simulink library "HEMERO"  (Simulink 3.00)
values from neighbouring files (symbols this model uses):
  K1 = 0.5    [ejh64.m]    (also in ejh65.m)
  K2 = 0.8    [ejh64.m]    (also in ejh65.m)
  x_camino = 0:0.01:10    [ejh64.m]    (also in ejh65.m)
  y_camino = x_camino.^2    [ejh64.m]    (also in ejh65.m)
undefined symbols (not defined in the file or in its folder): magnitude, nonlinear
libraries: simulink_extras x12, HEMERO x9, simulink3 x6, dspstat x4
(part 9 of 9)

== system HEMERO/Robots móviles/Control de robots móviles/Métodos basados en Teoría de Control/Seguimiento de caminos/Ejemplos/Ejemplo H.6.4/Seguimiento de caminos (control lineal)/Cálculo de parámetros/Subsystem/Parametros de Curvatura/coordenada x c. curvatura ==
  x_1 : Inport  Port=1  PortWidth=-1  SampleTime=-1  DataType=auto
      settings: SignalType=auto
  x_2 : Inport  Port=2  PortWidth=-1  SampleTime=-1  DataType=auto
      settings: SignalType=auto
  x_3 : Inport  Port=3  PortWidth=-1  SampleTime=-1  DataType=auto
      settings: SignalType=auto
  y_1 : Inport  Port=4  PortWidth=-1  SampleTime=-1  DataType=auto
      settings: SignalType=auto
  y_2 : Inport  Port=5  PortWidth=-1  SampleTime=-1  DataType=auto
      settings: SignalType=auto
  y_3 : Inport  Port=6  PortWidth=-1  SampleTime=-1  DataType=auto
      settings: SignalType=auto
  Constant : Constant  Value=0.00000001
  Math Function : Math  Operator=reciprocal  OutputSignalType=auto
  Product{,1..4} (5 alike) : Product  Inputs=2  SaturateOnIntegerOverflow=on
  Sum : Sum  Inputs=+-  SaturateOnIntegerOverflow=on
  Sum1 : Sum  Inputs=+-  SaturateOnIntegerOverflow=on
  Switch : Switch  Threshold=0.00000001
  bloque_1 : Subsystem
  bloque_2 : Subsystem
  x_g : Outport  Port=1  InitialOutput=0
  wires:
  Switch/1 -> Math Function/1
  Constant/1 -> Switch/3
  Sum1/1 -> Switch/1, Switch/2
  Product4/1 -> x_g/1
  Product/1 -> Sum/1
  Product1/1 -> Sum/2
  Product2/1 -> Sum1/1
  Product3/1 -> Sum1/2
  Math Function/1 -> Product4/2
  bloque_1/3(c_1) -> Product/2
  bloque_2/3(c_2) -> Product1/2
  bloque_2/2(beta_2) -> Product/1, Product2/2
  bloque_1/1(alfa_1) -> Product2/1
  bloque_1/2(beta_1) -> Product1/1, Product3/1
  bloque_2/1(alfa_2) -> Product3/2
  x_1/1 -> bloque_1/1(x1)
  x_2/1 -> bloque_1/2(x2), bloque_2/1(x2)
  y_1/1 -> bloque_1/3(y1)
  x_3/1 -> bloque_2/2(x3)
  y_2/1 -> bloque_2/3(y2), bloque_1/4(y2)
  y_3/1 -> bloque_2/4(y3)
  Sum/1 -> Product4/1

== system HEMERO/Robots móviles/Control de robots móviles/Métodos basados en Teoría de Control/Seguimiento de caminos/Ejemplos/Ejemplo H.6.4/Seguimiento de caminos (control lineal)/Cálculo de parámetros/Subsystem/Parametros de Curvatura/coordenada y c. curvatura ==
  x_1 : Inport  Port=1  PortWidth=-1  SampleTime=-1  DataType=auto
      settings: SignalType=auto
  x_2 : Inport  Port=2  PortWidth=-1  SampleTime=-1  DataType=auto
      settings: SignalType=auto
  x_3 : Inport  Port=3  PortWidth=-1  SampleTime=-1  DataType=auto
      settings: SignalType=auto
  y_1 : Inport  Port=4  PortWidth=-1  SampleTime=-1  DataType=auto
      settings: SignalType=auto
  y_2 : Inport  Port=5  PortWidth=-1  SampleTime=-1  DataType=auto
      settings: SignalType=auto
  y_3 : Inport  Port=6  PortWidth=-1  SampleTime=-1  DataType=auto
      settings: SignalType=auto
  Constant : Constant  Value=0.00000001
  Math Function : Math  Operator=reciprocal  OutputSignalType=auto
  Product{,1..4} (5 alike) : Product  Inputs=2  SaturateOnIntegerOverflow=on
  Sum : Sum  Inputs=+-  SaturateOnIntegerOverflow=on
  Sum1 : Sum  Inputs=+-  SaturateOnIntegerOverflow=on
  Switch : Switch  Threshold=0.00000001
  bloque_1 : Subsystem
  bloque_2 : Subsystem
  y_g : Outport  Port=1  InitialOutput=0
  wires:
  Constant/1 -> Switch/3
  Sum1/1 -> Switch/1, Switch/2
  Switch/1 -> Math Function/1
  Math Function/1 -> Product4/2
  Product4/1 -> y_g/1
  bloque_2/3(c_2) -> Product/2
  bloque_1/3(c_1) -> Product1/1
  bloque_1/1(alfa_1) -> Product/1, Product2/1
  bloque_2/2(beta_2) -> Product2/2
  bloque_1/2(beta_1) -> Product3/2
  bloque_2/1(alfa_2) -> Product1/2, Product3/1
  Product/1 -> Sum/1
  Product1/1 -> Sum/2
  Product2/1 -> Sum1/1
  Product3/1 -> Sum1/2
  x_1/1 -> bloque_1/1(x1)
  x_2/1 -> bloque_1/2(x2), bloque_2/1(x2)
  y_1/1 -> bloque_1/3(y1)
  x_3/1 -> bloque_2/2(x3)
  y_2/1 -> bloque_2/3(y2), bloque_1/4(y2)
  y_3/1 -> bloque_2/4(y3)
  Sum/1 -> Product4/1

== system HEMERO/Robots móviles/Control de robots móviles/Métodos basados en Teoría de Control/Seguimiento de caminos/Ejemplos/Ejemplo H.6.5/Seguimiento de caminos (control no lineal)/Cálculo de parámetros/Subsystem/Parametros de Curvatura/Radio de  Curvatura ==
  x_g : Inport  Port=1  PortWidth=-1  SampleTime=-1  DataType=auto
      settings: SignalType=auto
  x_1 : Inport  Port=2  PortWidth=-1  SampleTime=-1  DataType=auto
      settings: SignalType=auto
  y_g : Inport  Port=3  PortWidth=-1  SampleTime=-1  DataType=auto
      settings: SignalType=auto
  y_1 : Inport  Port=4  PortWidth=-1  SampleTime=-1  DataType=auto
      settings: SignalType=auto
  Math Function : Math  Operator=square  OutputSignalType=auto
  Math Function1 : Math  Operator=sqrt  OutputSignalType=auto
  Math Function2 : Math  Operator=square  OutputSignalType=auto
  Sum : Sum  Inputs=+-  SaturateOnIntegerOverflow=on
  Sum1 : Sum  Inputs=+-  SaturateOnIntegerOverflow=on
  Sum2 : Sum  Inputs=++  SaturateOnIntegerOverflow=on
  R_c : Outport  Port=1  InitialOutput=0
  wires:
  Math Function1/1 -> R_c/1
  Sum2/1 -> Math Function1/1
  Math Function2/1 -> Sum2/2
  Math Function/1 -> Sum2/1
  Sum1/1 -> Math Function2/1
  Sum/1 -> Math Function/1
  y_g/1 -> Sum1/2
  y_1/1 -> Sum1/1
  x_1/1 -> Sum/1
  x_g/1 -> Sum/2

== system HEMERO/Robots móviles/Control de robots móviles/Métodos basados en Teoría de Control/Seguimiento de caminos/Ejemplos/Ejemplo H.6.5/Seguimiento de caminos (control no lineal)/Cálculo de parámetros/Subsystem/Parametros de Curvatura/coordenada x c. curvatura ==
  x_1 : Inport  Port=1  PortWidth=-1  SampleTime=-1  DataType=auto
      settings: SignalType=auto
  x_2 : Inport  Port=2  PortWidth=-1  SampleTime=-1  DataType=auto
      settings: SignalType=auto
  x_3 : Inport  Port=3  PortWidth=-1  SampleTime=-1  DataType=auto
      settings: SignalType=auto
  y_1 : Inport  Port=4  PortWidth=-1  SampleTime=-1  DataType=auto
      settings: SignalType=auto
  y_2 : Inport  Port=5  PortWidth=-1  SampleTime=-1  DataType=auto
      settings: SignalType=auto
  y_3 : Inport  Port=6  PortWidth=-1  SampleTime=-1  DataType=auto
      settings: SignalType=auto
  Constant : Constant  Value=0.00000001
  Math Function : Math  Operator=reciprocal  OutputSignalType=auto
  Product{,1..4} (5 alike) : Product  Inputs=2  SaturateOnIntegerOverflow=on
  Sum : Sum  Inputs=+-  SaturateOnIntegerOverflow=on
  Sum1 : Sum  Inputs=+-  SaturateOnIntegerOverflow=on
  Switch : Switch  Threshold=0.00000001
  bloque_1 : Subsystem
  bloque_2 : Subsystem
  x_g : Outport  Port=1  InitialOutput=0
  wires:
  Switch/1 -> Math Function/1
  Constant/1 -> Switch/3
  Sum1/1 -> Switch/1, Switch/2
  Product4/1 -> x_g/1
  Product/1 -> Sum/1
  Product1/1 -> Sum/2
  Product2/1 -> Sum1/1
  Product3/1 -> Sum1/2
  Math Function/1 -> Product4/2
  bloque_1/3(c_1) -> Product/2
  bloque_2/3(c_2) -> Product1/2
  bloque_2/2(beta_2) -> Product/1, Product2/2
  bloque_1/1(alfa_1) -> Product2/1
  bloque_1/2(beta_1) -> Product1/1, Product3/1
  bloque_2/1(alfa_2) -> Product3/2
  x_1/1 -> bloque_1/1(x1)
  x_2/1 -> bloque_1/2(x2), bloque_2/1(x2)
  y_1/1 -> bloque_1/3(y1)
  x_3/1 -> bloque_2/2(x3)
  y_2/1 -> bloque_2/3(y2), bloque_1/4(y2)
  y_3/1 -> bloque_2/4(y3)
  Sum/1 -> Product4/1

== system HEMERO/Robots móviles/Control de robots móviles/Métodos basados en Teoría de Control/Seguimiento de caminos/Ejemplos/Ejemplo H.6.5/Seguimiento de caminos (control no lineal)/Cálculo de parámetros/Subsystem/Parametros de Curvatura/coordenada y c. curvatura ==
  x_1 : Inport  Port=1  PortWidth=-1  SampleTime=-1  DataType=auto
      settings: SignalType=auto
  x_2 : Inport  Port=2  PortWidth=-1  SampleTime=-1  DataType=auto
      settings: SignalType=auto
  x_3 : Inport  Port=3  PortWidth=-1  SampleTime=-1  DataType=auto
      settings: SignalType=auto
  y_1 : Inport  Port=4  PortWidth=-1  SampleTime=-1  DataType=auto
      settings: SignalType=auto
  y_2 : Inport  Port=5  PortWidth=-1  SampleTime=-1  DataType=auto
      settings: SignalType=auto
  y_3 : Inport  Port=6  PortWidth=-1  SampleTime=-1  DataType=auto
      settings: SignalType=auto
  Constant : Constant  Value=0.00000001
  Math Function : Math  Operator=reciprocal  OutputSignalType=auto
  Product{,1..4} (5 alike) : Product  Inputs=2  SaturateOnIntegerOverflow=on
  Sum : Sum  Inputs=+-  SaturateOnIntegerOverflow=on
  Sum1 : Sum  Inputs=+-  SaturateOnIntegerOverflow=on
  Switch : Switch  Threshold=0.00000001
  bloque_1 : Subsystem
  bloque_2 : Subsystem
  y_g : Outport  Port=1  InitialOutput=0
  wires:
  Constant/1 -> Switch/3
  Sum1/1 -> Switch/1, Switch/2
  Switch/1 -> Math Function/1
  Math Function/1 -> Product4/2
  Product4/1 -> y_g/1
  bloque_2/3(c_2) -> Product/2
  bloque_1/3(c_1) -> Product1/1
  bloque_1/1(alfa_1) -> Product/1, Product2/1
  bloque_2/2(beta_2) -> Product2/2
  bloque_1/2(beta_1) -> Product3/2
  bloque_2/1(alfa_2) -> Product1/2, Product3/1
  Product/1 -> Sum/1
  Product1/1 -> Sum/2
  Product2/1 -> Sum1/1
  Product3/1 -> Sum1/2
  x_1/1 -> bloque_1/1(x1)
  x_2/1 -> bloque_1/2(x2), bloque_2/1(x2)
  y_1/1 -> bloque_1/3(y1)
  x_3/1 -> bloque_2/2(x3)
  y_2/1 -> bloque_2/3(y2), bloque_1/4(y2)
  y_3/1 -> bloque_2/4(y3)
  Sum/1 -> Product4/1

== system HEMERO/Robots móviles/Control de robots móviles/Métodos basados en Teoría de Control/Seguimiento de caminos/Ejemplos/Ejemplo H.6.4/Seguimiento de caminos (control lineal)/Cálculo de parámetros/Subsystem/Parametros de Curvatura/coordenada x c. curvatura/bloque_1 ==
  x1 : Inport  Port=1  PortWidth=-1  SampleTime=-1  DataType=auto
      settings: SignalType=auto
  x2 : Inport  Port=2  PortWidth=-1  SampleTime=-1  DataType=auto
      settings: SignalType=auto
  y1 : Inport  Port=3  PortWidth=-1  SampleTime=-1  DataType=auto
      settings: SignalType=auto
  y2 : Inport  Port=4  PortWidth=-1  SampleTime=-1  DataType=auto
      settings: SignalType=auto
  Gain : Gain  Gain=0.5  SaturateOnIntegerOverflow=on
  Math Function{,1..3} (4 alike) : Math  Operator=square  OutputSignalType=auto
  Sum : Sum  Inputs=-+  SaturateOnIntegerOverflow=on
  Sum1 : Sum  Inputs=-+  SaturateOnIntegerOverflow=on
  Sum2 : Sum  Inputs=-+-+  SaturateOnIntegerOverflow=on
  alfa_1 : Outport  Port=1  InitialOutput=0
  beta_1 : Outport  Port=2  InitialOutput=0
  c_1 : Outport  Port=3  InitialOutput=0
  wires:
  Sum/1 -> alfa_1/1
  Sum1/1 -> beta_1/1
  x1/1 -> Sum/1, Math Function/1
  x2/1 -> Sum/2, Math Function1/1
  y1/1 -> Sum1/1, Math Function2/1
  y2/1 -> Sum1/2, Math Function3/1
  Math Function/1 -> Sum2/1
  Math Function1/1 -> Sum2/2
  Math Function2/1 -> Sum2/3
  Math Function3/1 -> Sum2/4
  Sum2/1 -> Gain/1
  Gain/1 -> c_1/1

== system HEMERO/Robots móviles/Control de robots móviles/Métodos basados en Teoría de Control/Seguimiento de caminos/Ejemplos/Ejemplo H.6.4/Seguimiento de caminos (control lineal)/Cálculo de parámetros/Subsystem/Parametros de Curvatura/coordenada x c. curvatura/bloque_2 ==
  x2 : Inport  Port=1  PortWidth=-1  SampleTime=-1  DataType=auto
      settings: SignalType=auto
  x3 : Inport  Port=2  PortWidth=-1  SampleTime=-1  DataType=auto
      settings: SignalType=auto
  y2 : Inport  Port=3  PortWidth=-1  SampleTime=-1  DataType=auto
      settings: SignalType=auto
  y3 : Inport  Port=4  PortWidth=-1  SampleTime=-1  DataType=auto
      settings: SignalType=auto
  Gain : Gain  Gain=0.5  SaturateOnIntegerOverflow=on
  Math Function{,1..3} (4 alike) : Math  Operator=square  OutputSignalType=auto
  Sum : Sum  Inputs=-+  SaturateOnIntegerOverflow=on
  Sum1 : Sum  Inputs=-+  SaturateOnIntegerOverflow=on
  Sum2 : Sum  Inputs=-+-+  SaturateOnIntegerOverflow=on
  alfa_2 : Outport  Port=1  InitialOutput=0
  beta_2 : Outport  Port=2  InitialOutput=0
  c_2 : Outport  Port=3  InitialOutput=0
  wires:
  Sum/1 -> alfa_2/1
  Sum1/1 -> beta_2/1
  x2/1 -> Sum/1, Math Function/1
  x3/1 -> Sum/2, Math Function1/1
  y2/1 -> Sum1/1, Math Function2/1
  y3/1 -> Sum1/2, Math Function3/1
  Math Function/1 -> Sum2/1
  Math Function1/1 -> Sum2/2
  Math Function2/1 -> Sum2/3
  Math Function3/1 -> Sum2/4
  Sum2/1 -> Gain/1
  Gain/1 -> c_2/1

== system HEMERO/Robots móviles/Control de robots móviles/Métodos basados en Teoría de Control/Seguimiento de caminos/Ejemplos/Ejemplo H.6.4/Seguimiento de caminos (control lineal)/Cálculo de parámetros/Subsystem/Parametros de Curvatura/coordenada y c. curvatura/bloque_1 ==
  x1 : Inport  Port=1  PortWidth=-1  SampleTime=-1  DataType=auto
      settings: SignalType=auto
  x2 : Inport  Port=2  PortWidth=-1  SampleTime=-1  DataType=auto
      settings: SignalType=auto
  y1 : Inport  Port=3  PortWidth=-1  SampleTime=-1  DataType=auto
      settings: SignalType=auto
  y2 : Inport  Port=4  PortWidth=-1  SampleTime=-1  DataType=auto
      settings: SignalType=auto
  Gain : Gain  Gain=0.5  SaturateOnIntegerOverflow=on
  Math Function{,1..3} (4 alike) : Math  Operator=square  OutputSignalType=auto
  Sum : Sum  Inputs=-+  SaturateOnIntegerOverflow=on
  Sum1 : Sum  Inputs=-+  SaturateOnIntegerOverflow=on
  Sum2 : Sum  Inputs=-+-+  SaturateOnIntegerOverflow=on
  alfa_1 : Outport  Port=1  InitialOutput=0
  beta_1 : Outport  Port=2  InitialOutput=0
  c_1 : Outport  Port=3  InitialOutput=0
  wires:
  Sum/1 -> alfa_1/1
  Sum1/1 -> beta_1/1
  x1/1 -> Sum/1, Math Function/1
  x2/1 -> Sum/2, Math Function1/1
  y1/1 -> Sum1/1, Math Function2/1
  y2/1 -> Sum1/2, Math Function3/1
  Math Function/1 -> Sum2/1
  Math Function1/1 -> Sum2/2
  Math Function2/1 -> Sum2/3
  Math Function3/1 -> Sum2/4
  Sum2/1 -> Gain/1
  Gain/1 -> c_1/1

== system HEMERO/Robots móviles/Control de robots móviles/Métodos basados en Teoría de Control/Seguimiento de caminos/Ejemplos/Ejemplo H.6.4/Seguimiento de caminos (control lineal)/Cálculo de parámetros/Subsystem/Parametros de Curvatura/coordenada y c. curvatura/bloque_2 ==
  x2 : Inport  Port=1  PortWidth=-1  SampleTime=-1  DataType=auto
      settings: SignalType=auto
  x3 : Inport  Port=2  PortWidth=-1  SampleTime=-1  DataType=auto
      settings: SignalType=auto
  y2 : Inport  Port=3  PortWidth=-1  SampleTime=-1  DataType=auto
      settings: SignalType=auto
  y3 : Inport  Port=4  PortWidth=-1  SampleTime=-1  DataType=auto
      settings: SignalType=auto
  Gain : Gain  Gain=0.5  SaturateOnIntegerOverflow=on
  Math Function{,1..3} (4 alike) : Math  Operator=square  OutputSignalType=auto
  Sum : Sum  Inputs=-+  SaturateOnIntegerOverflow=on
  Sum1 : Sum  Inputs=-+  SaturateOnIntegerOverflow=on
  Sum2 : Sum  Inputs=-+-+  SaturateOnIntegerOverflow=on
  alfa_2 : Outport  Port=1  InitialOutput=0
  beta_2 : Outport  Port=2  InitialOutput=0
  c_2 : Outport  Port=3  InitialOutput=0
  wires:
  Sum/1 -> alfa_2/1
  Sum1/1 -> beta_2/1
  x2/1 -> Sum/1, Math Function/1
  x3/1 -> Sum/2, Math Function1/1
  y2/1 -> Sum1/1, Math Function2/1
  y3/1 -> Sum1/2, Math Function3/1
  Math Function/1 -> Sum2/1
  Math Function1/1 -> Sum2/2
  Math Function2/1 -> Sum2/3
  Math Function3/1 -> Sum2/4
  Sum2/1 -> Gain/1
  Gain/1 -> c_2/1

== system HEMERO/Robots móviles/Control de robots móviles/Métodos basados en Teoría de Control/Seguimiento de caminos/Ejemplos/Ejemplo H.6.5/Seguimiento de caminos (control no lineal)/Cálculo de parámetros/Subsystem/Parametros de Curvatura/coordenada x c. curvatura/bloque_1 ==
  x1 : Inport  Port=1  PortWidth=-1  SampleTime=-1  DataType=auto
      settings: SignalType=auto
  x2 : Inport  Port=2  PortWidth=-1  SampleTime=-1  DataType=auto
      settings: SignalType=auto
  y1 : Inport  Port=3  PortWidth=-1  SampleTime=-1  DataType=auto
      settings: SignalType=auto
  y2 : Inport  Port=4  PortWidth=-1  SampleTime=-1  DataType=auto
      settings: SignalType=auto
  Gain : Gain  Gain=0.5  SaturateOnIntegerOverflow=on
  Math Function{,1..3} (4 alike) : Math  Operator=square  OutputSignalType=auto
  Sum : Sum  Inputs=-+  SaturateOnIntegerOverflow=on
  Sum1 : Sum  Inputs=-+  SaturateOnIntegerOverflow=on
  Sum2 : Sum  Inputs=-+-+  SaturateOnIntegerOverflow=on
  alfa_1 : Outport  Port=1  InitialOutput=0
  beta_1 : Outport  Port=2  InitialOutput=0
  c_1 : Outport  Port=3  InitialOutput=0
  wires:
  Sum/1 -> alfa_1/1
  Sum1/1 -> beta_1/1
  x1/1 -> Sum/1, Math Function/1
  x2/1 -> Sum/2, Math Function1/1
  y1/1 -> Sum1/1, Math Function2/1
  y2/1 -> Sum1/2, Math Function3/1
  Math Function/1 -> Sum2/1
  Math Function1/1 -> Sum2/2
  Math Function2/1 -> Sum2/3
  Math Function3/1 -> Sum2/4
  Sum2/1 -> Gain/1
  Gain/1 -> c_1/1

== system HEMERO/Robots móviles/Control de robots móviles/Métodos basados en Teoría de Control/Seguimiento de caminos/Ejemplos/Ejemplo H.6.5/Seguimiento de caminos (control no lineal)/Cálculo de parámetros/Subsystem/Parametros de Curvatura/coordenada x c. curvatura/bloque_2 ==
  x2 : Inport  Port=1  PortWidth=-1  SampleTime=-1  DataType=auto
      settings: SignalType=auto
  x3 : Inport  Port=2  PortWidth=-1  SampleTime=-1  DataType=auto
      settings: SignalType=auto
  y2 : Inport  Port=3  PortWidth=-1  SampleTime=-1  DataType=auto
      settings: SignalType=auto
  y3 : Inport  Port=4  PortWidth=-1  SampleTime=-1  DataType=auto
      settings: SignalType=auto
  Gain : Gain  Gain=0.5  SaturateOnIntegerOverflow=on
  Math Function{,1..3} (4 alike) : Math  Operator=square  OutputSignalType=auto
  Sum : Sum  Inputs=-+  SaturateOnIntegerOverflow=on
  Sum1 : Sum  Inputs=-+  SaturateOnIntegerOverflow=on
  Sum2 : Sum  Inputs=-+-+  SaturateOnIntegerOverflow=on
  alfa_2 : Outport  Port=1  InitialOutput=0
  beta_2 : Outport  Port=2  InitialOutput=0
  c_2 : Outport  Port=3  InitialOutput=0
  wires:
  Sum/1 -> alfa_2/1
  Sum1/1 -> beta_2/1
  x2/1 -> Sum/1, Math Function/1
  x3/1 -> Sum/2, Math Function1/1
  y2/1 -> Sum1/1, Math Function2/1
  y3/1 -> Sum1/2, Math Function3/1
  Math Function/1 -> Sum2/1
  Math Function1/1 -> Sum2/2
  Math Function2/1 -> Sum2/3
  Math Function3/1 -> Sum2/4
  Sum2/1 -> Gain/1
  Gain/1 -> c_2/1

== system HEMERO/Robots móviles/Control de robots móviles/Métodos basados en Teoría de Control/Seguimiento de caminos/Ejemplos/Ejemplo H.6.5/Seguimiento de caminos (control no lineal)/Cálculo de parámetros/Subsystem/Parametros de Curvatura/coordenada y c. curvatura/bloque_1 ==
  x1 : Inport  Port=1  PortWidth=-1  SampleTime=-1  DataType=auto
      settings: SignalType=auto
  x2 : Inport  Port=2  PortWidth=-1  SampleTime=-1  DataType=auto
      settings: SignalType=auto
  y1 : Inport  Port=3  PortWidth=-1  SampleTime=-1  DataType=auto
      settings: SignalType=auto
  y2 : Inport  Port=4  PortWidth=-1  SampleTime=-1  DataType=auto
      settings: SignalType=auto
  Gain : Gain  Gain=0.5  SaturateOnIntegerOverflow=on
  Math Function{,1..3} (4 alike) : Math  Operator=square  OutputSignalType=auto
  Sum : Sum  Inputs=-+  SaturateOnIntegerOverflow=on
  Sum1 : Sum  Inputs=-+  SaturateOnIntegerOverflow=on
  Sum2 : Sum  Inputs=-+-+  SaturateOnIntegerOverflow=on
  alfa_1 : Outport  Port=1  InitialOutput=0
  beta_1 : Outport  Port=2  InitialOutput=0
  c_1 : Outport  Port=3  InitialOutput=0
  wires:
  Sum/1 -> alfa_1/1
  Sum1/1 -> beta_1/1
  x1/1 -> Sum/1, Math Function/1
  x2/1 -> Sum/2, Math Function1/1
  y1/1 -> Sum1/1, Math Function2/1
  y2/1 -> Sum1/2, Math Function3/1
  Math Function/1 -> Sum2/1
  Math Function1/1 -> Sum2/2
  Math Function2/1 -> Sum2/3
  Math Function3/1 -> Sum2/4
  Sum2/1 -> Gain/1
  Gain/1 -> c_1/1

== system HEMERO/Robots móviles/Control de robots móviles/Métodos basados en Teoría de Control/Seguimiento de caminos/Ejemplos/Ejemplo H.6.5/Seguimiento de caminos (control no lineal)/Cálculo de parámetros/Subsystem/Parametros de Curvatura/coordenada y c. curvatura/bloque_2 ==
  x2 : Inport  Port=1  PortWidth=-1  SampleTime=-1  DataType=auto
      settings: SignalType=auto
  x3 : Inport  Port=2  PortWidth=-1  SampleTime=-1  DataType=auto
      settings: SignalType=auto
  y2 : Inport  Port=3  PortWidth=-1  SampleTime=-1  DataType=auto
      settings: SignalType=auto
  y3 : Inport  Port=4  PortWidth=-1  SampleTime=-1  DataType=auto
      settings: SignalType=auto
  Gain : Gain  Gain=0.5  SaturateOnIntegerOverflow=on
  Math Function{,1..3} (4 alike) : Math  Operator=square  OutputSignalType=auto
  Sum : Sum  Inputs=-+  SaturateOnIntegerOverflow=on
  Sum1 : Sum  Inputs=-+  SaturateOnIntegerOverflow=on
  Sum2 : Sum  Inputs=-+-+  SaturateOnIntegerOverflow=on
  alfa_2 : Outport  Port=1  InitialOutput=0
  beta_2 : Outport  Port=2  InitialOutput=0
  c_2 : Outport  Port=3  InitialOutput=0
  wires:
  Sum/1 -> alfa_2/1
  Sum1/1 -> beta_2/1
  x2/1 -> Sum/1, Math Function/1
  x3/1 -> Sum/2, Math Function1/1
  y2/1 -> Sum1/1, Math Function2/1
  y3/1 -> Sum1/2, Math Function3/1
  Math Function/1 -> Sum2/1
  Math Function1/1 -> Sum2/2
  Math Function2/1 -> Sum2/3
  Math Function3/1 -> Sum2/4
  Sum2/1 -> Gain/1
  Gain/1 -> c_2/1
